simulink model "CARTESIAN_SPACE"  (R2018b)
settings: Solver=FixedStepAuto  StartTime=0.0  StopTime=25  FixedStep=0.01  RelTol=1e-3
model workspace: external: MATLAB File D:\OneDrive\STUDY\RIC LAB\PROJECT 6DOF\CODE\CODE 6DOF\06_TRAJECTORY PLANNING\02\ROBOT_DataFile.m (data not in the file)
undefined symbols (not defined in the file or in its folder): circle, smiData, X, Y, Z
libraries: sm_lib x38, nesl_utility x16, simulink_extras x1
(part 1 of 2)
settings Model: Creator=TMP  LastModifiedBy=TMP

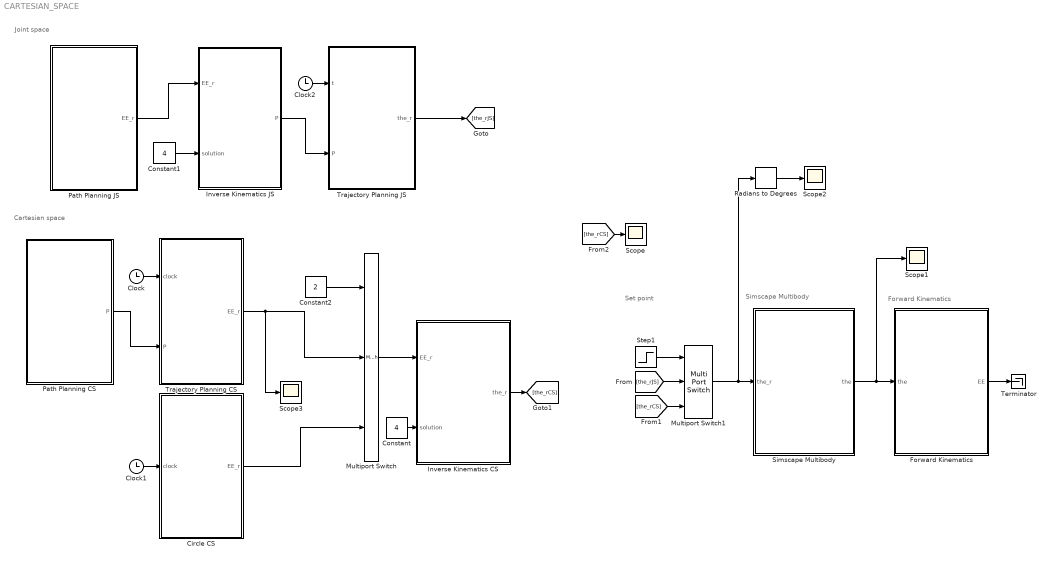
== system CARTESIAN_SPACE ==
  note: Set point
  note: Cartesian space
  note: Joint space
  note: Forward Kinematics
  note: Simscape Multibody
  Circle CS : MATLAB Function  TreatAsAtomicUnit=on
  Clock : Clock
  Clock1 : Clock
  Clock2 : Clock
  Constant : Constant  Value=4
  Constant1 : Constant  Value=4
  Constant2 : Constant  Value=2
  Forward Kinematics : MATLAB Function  TreatAsAtomicUnit=on
  Inverse Kinematics CS : MATLAB Function  TreatAsAtomicUnit=on
  Inverse Kinematics JS : MATLAB Function  TreatAsAtomicUnit=on
  Multiport Switch : MultiPortSwitch  Inputs=2
  Multiport Switch1 : MultiPortSwitch  Inputs=2
  Path Planning CS : Subsystem
  Path Planning JS : Subsystem
  Radians to Degrees : simulink_extras/Transformations/Radians to Degrees
  Scope{,1..3} (4 alike) : Scope
  Simscape Multibody : Subsystem
  Step1 : Step  Time=5  Before=1  After=2  SampleTime=0
  Terminator : Terminator
  Trajectory Planning CS : MATLAB Function  TreatAsAtomicUnit=on
  Trajectory Planning JS : MATLAB Function  TreatAsAtomicUnit=on
  wires:
  Clock1/1 -> Circle CS/1(clock)
  Circle CS/1(EE_r) -> Multiport Switch/3
  Constant/1 -> Inverse Kinematics CS/2(solution)
  Simscape Multibody/1(the) -> Scope1/1, Forward Kinematics/1(the)
  Multiport Switch/1 -> Inverse Kinematics CS/1(EE_r)
  Clock/1 -> Trajectory Planning CS/1(clock)
  Trajectory Planning CS/1(EE_r) -> Scope3/1, Multiport Switch/2
  Path Planning CS/1(P) -> Trajectory Planning CS/2(P)
  Constant2/1 -> Multiport Switch/1
  Clock2/1 -> Trajectory Planning JS/1(t)
  Path Planning JS/1(EE_r) -> Inverse Kinematics JS/1(EE_r)
  Constant1/1 -> Inverse Kinematics JS/2(solution)
  Inverse Kinematics JS/1(P) -> Trajectory Planning JS/2(P)
  Step1/1 -> Multiport Switch1/1
  Trajectory Planning JS/1(the_r) -> [the_rJS]
  Inverse Kinematics CS/1(the_r) -> [the_rCS]
  [the_rJS] -> Multiport Switch1/2
  [the_rCS] -> Multiport Switch1/3
  Forward Kinematics/1(EE) -> Terminator/1
  Multiport Switch1/1 -> Radians to Degrees/1, Simscape Multibody/1(the_r)
  [the_rCS] -> Scope/1
  Radians to Degrees/1 -> Scope2/1

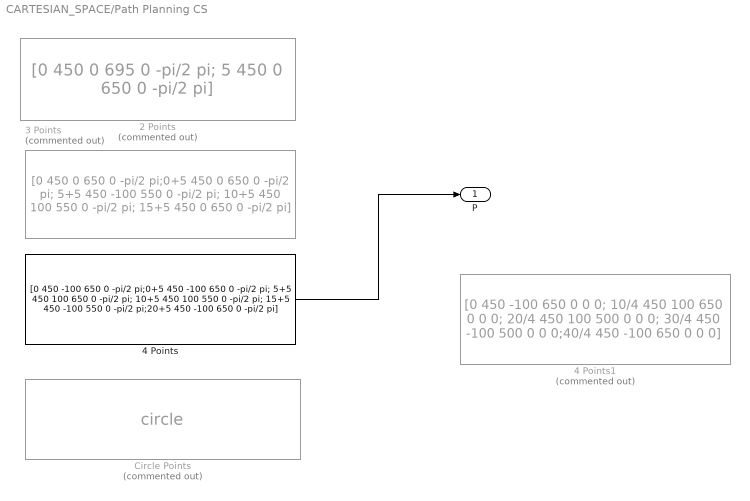
== system CARTESIAN_SPACE/Path Planning CS ==
  2 Points : Constant  Commented=on  Value=[0 450 0 695 0 -pi/2 pi; 5 450 0 650 0 -pi/2 pi]
  3 Points : Constant  Commented=on  Value=[0 450 0 650 0 -pi/2 pi;0+5 450 0 650 0 -pi/2 pi; 5+5 450 -100 550 0 -pi/2 pi; 10+5 450 100 550 0 -pi/2 pi; 15+5 450 0 650 0 -pi/2 pi]
  4 Points : Constant  Value=[0 450 -100 650 0 -pi/2 pi;0+5 450 -100 650 0 -pi/2 pi; 5+5 450 100 650 0 -pi/2 pi; 10+5 450 100 550 0 -pi/2 pi; 15+5 450 -100 550 0 -pi/2 pi;20+5 450 -100 650 0 -pi/2 pi]
  4 Points1 : Constant  Commented=on  Value=[0 450 -100 650 0 0 0; 10/4 450 100 650 0 0 0; 20/4 450 100 500 0 0 0; 30/4 450 -100 500 0 0 0;40/4 450 -100 650 0 0 0]
  Circle Points : Constant  Commented=on  Value=circle
  P : Outport
  wires:
  4 Points/1 -> P/1

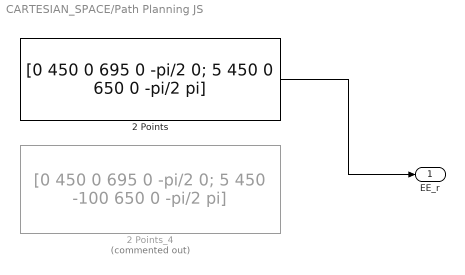
== system CARTESIAN_SPACE/Path Planning JS ==
  2 Points : Constant  Value=[0 450 0 695 0 -pi/2 0; 5 450 0 650 0 -pi/2 pi]
  2 Points_4 : Constant  Commented=on  Value=[0 450 0 695 0 -pi/2 0; 5 450 -100 650 0 -pi/2 pi]
  EE_r : Outport
  wires:
  2 Points/1 -> EE_r/1

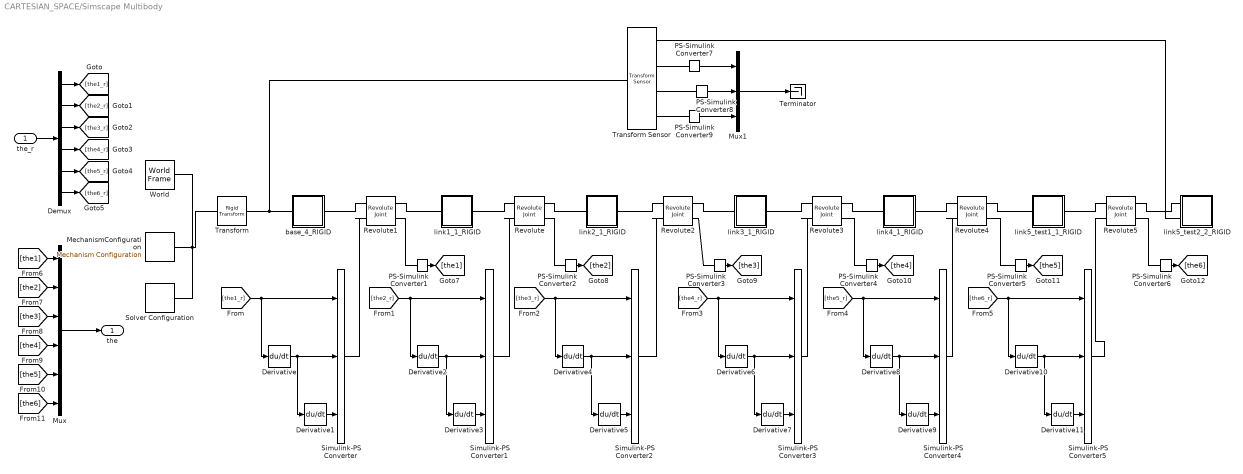
== system CARTESIAN_SPACE/Simscape Multibody ==
  the_r : Inport
  Demux : Demux  Outputs=6
  Derivative{,1..11} (12 alike) : Derivative
  MechanismConfiguration : sm_lib/Utilities/Mechanism Configuration  UniformGravity=Constant  GravityVector=[0 -9.80665 0]  GravityUnits=m/s^2  LinearizationDelta=0.001
  Mux : Mux  Inputs=6
  Mux1 : Mux  Inputs=3
  PS-Simulink Converter{1..9} (9 alike) : nesl_utility/PS-Simulink Converter  PhysicalDomain=network_engine_domain  SubClassName=ps_output  LeftPortType=input  RightPortType=output  PseudoPeriodic=off  Frequencies=[]  Unit=1  AffineConversion=off
  Revolute : sm_lib/Joints/Revolute Joint  SenseConstraintForce=off  SenseConstraintForceX=off  SenseConstraintForceY=off  SenseConstraintForceZ=off  SenseConstraintTorque=off  SenseConstraintTorqueX=off  SenseConstraintTorqueY=off  SenseConstraintTorqueZ=off  SenseTotalForce=off  SenseTotalForceX=off  SenseTotalForceY=off  SenseTotalForceZ=off  SenseTotalTorque=off  SenseTotalTorqueX=off  SenseTotalTorqueY=off  SenseTotalTorqueZ=off  CompositeWrenchDir=FollowerOnBase  CompositeWrenchFrame=BaseFrame  EquilibriumPosition=0  EquilibriumPositionUnits=rad  SpringStiffness=0  SpringStiffnessUnits=N*m/rad  DampingCoefficient=0  DampingCoefficientUnits=N*m/(rad/s)  TorqueActuationMode=ComputedTorque  MotionActuationMode=InputMotion  SensePosition=on  SenseVelocity=off  SenseAcceleration=off  SenseTorqueForce=off  PositionTargetSpecify=on  PositionTargetPriority=Low  PositionTargetValue=smiData.RevoluteJoint(1).Rz.Pos  PositionTargetValueUnits=deg  VelocityTargetSpecify=off  VelocityTargetPriority=High  VelocityTargetValue=0  VelocityTargetValueUnits=deg/s
  Revolute1 : sm_lib/Joints/Revolute Joint  SenseConstraintForce=off  SenseConstraintForceX=off  SenseConstraintForceY=off  SenseConstraintForceZ=off  SenseConstraintTorque=off  SenseConstraintTorqueX=off  SenseConstraintTorqueY=off  SenseConstraintTorqueZ=off  SenseTotalForce=off  SenseTotalForceX=off  SenseTotalForceY=off  SenseTotalForceZ=off  SenseTotalTorque=off  SenseTotalTorqueX=off  SenseTotalTorqueY=off  SenseTotalTorqueZ=off  CompositeWrenchDir=FollowerOnBase  CompositeWrenchFrame=BaseFrame  EquilibriumPosition=0  EquilibriumPositionUnits=rad  SpringStiffness=0  SpringStiffnessUnits=N*m/rad  DampingCoefficient=0  DampingCoefficientUnits=N*m/(rad/s)  TorqueActuationMode=ComputedTorque  MotionActuationMode=InputMotion  SensePosition=on  SenseVelocity=off  SenseAcceleration=off  SenseTorqueForce=off  PositionTargetSpecify=on  PositionTargetPriority=Low  PositionTargetValue=smiData.RevoluteJoint(2).Rz.Pos  PositionTargetValueUnits=deg  VelocityTargetSpecify=off  VelocityTargetPriority=High  VelocityTargetValue=0  VelocityTargetValueUnits=deg/s
  Revolute2 : sm_lib/Joints/Revolute Joint  SenseConstraintForce=off  SenseConstraintForceX=off  SenseConstraintForceY=off  SenseConstraintForceZ=off  SenseConstraintTorque=off  SenseConstraintTorqueX=off  SenseConstraintTorqueY=off  SenseConstraintTorqueZ=off  SenseTotalForce=off  SenseTotalForceX=off  SenseTotalForceY=off  SenseTotalForceZ=off  SenseTotalTorque=off  SenseTotalTorqueX=off  SenseTotalTorqueY=off  SenseTotalTorqueZ=off  CompositeWrenchDir=FollowerOnBase  CompositeWrenchFrame=BaseFrame  EquilibriumPosition=0  EquilibriumPositionUnits=rad  SpringStiffness=0  SpringStiffnessUnits=N*m/rad  DampingCoefficient=0  DampingCoefficientUnits=N*m/(rad/s)  TorqueActuationMode=ComputedTorque  MotionActuationMode=InputMotion  SensePosition=on  SenseVelocity=off  SenseAcceleration=off  SenseTorqueForce=off  PositionTargetSpecify=on  PositionTargetPriority=Low  PositionTargetValue=smiData.RevoluteJoint(3).Rz.Pos  PositionTargetValueUnits=deg  VelocityTargetSpecify=off  VelocityTargetPriority=High  VelocityTargetValue=0  VelocityTargetValueUnits=deg/s
  Revolute3 : sm_lib/Joints/Revolute Joint  SenseConstraintForce=off  SenseConstraintForceX=off  SenseConstraintForceY=off  SenseConstraintForceZ=off  SenseConstraintTorque=off  SenseConstraintTorqueX=off  SenseConstraintTorqueY=off  SenseConstraintTorqueZ=off  SenseTotalForce=off  SenseTotalForceX=off  SenseTotalForceY=off  SenseTotalForceZ=off  SenseTotalTorque=off  SenseTotalTorqueX=off  SenseTotalTorqueY=off  SenseTotalTorqueZ=off  CompositeWrenchDir=FollowerOnBase  CompositeWrenchFrame=BaseFrame  EquilibriumPosition=0  EquilibriumPositionUnits=rad  SpringStiffness=0  SpringStiffnessUnits=N*m/rad  DampingCoefficient=0  DampingCoefficientUnits=N*m/(rad/s)  TorqueActuationMode=ComputedTorque  MotionActuationMode=InputMotion  SensePosition=on  SenseVelocity=off  SenseAcceleration=off  SenseTorqueForce=off  PositionTargetSpecify=on  PositionTargetPriority=Low  PositionTargetValue=smiData.RevoluteJoint(4).Rz.Pos  PositionTargetValueUnits=deg  VelocityTargetSpecify=off  VelocityTargetPriority=High  VelocityTargetValue=0  VelocityTargetValueUnits=deg/s
  Revolute4 : sm_lib/Joints/Revolute Joint  SenseConstraintForce=off  SenseConstraintForceX=off  SenseConstraintForceY=off  SenseConstraintForceZ=off  SenseConstraintTorque=off  SenseConstraintTorqueX=off  SenseConstraintTorqueY=off  SenseConstraintTorqueZ=off  SenseTotalForce=off  SenseTotalForceX=off  SenseTotalForceY=off  SenseTotalForceZ=off  SenseTotalTorque=off  SenseTotalTorqueX=off  SenseTotalTorqueY=off  SenseTotalTorqueZ=off  CompositeWrenchDir=FollowerOnBase  CompositeWrenchFrame=BaseFrame  EquilibriumPosition=0  EquilibriumPositionUnits=rad  SpringStiffness=0  SpringStiffnessUnits=N*m/rad  DampingCoefficient=0  DampingCoefficientUnits=N*m/(rad/s)  TorqueActuationMode=ComputedTorque  MotionActuationMode=InputMotion  SensePosition=on  SenseVelocity=off  SenseAcceleration=off  SenseTorqueForce=off  PositionTargetSpecify=on  PositionTargetPriority=Low  PositionTargetValue=smiData.RevoluteJoint(5).Rz.Pos  PositionTargetValueUnits=deg  VelocityTargetSpecify=off  VelocityTargetPriority=High  VelocityTargetValue=0  VelocityTargetValueUnits=deg/s
  Revolute5 : sm_lib/Joints/Revolute Joint  SenseConstraintForce=off  SenseConstraintForceX=off  SenseConstraintForceY=off  SenseConstraintForceZ=off  SenseConstraintTorque=off  SenseConstraintTorqueX=off  SenseConstraintTorqueY=off  SenseConstraintTorqueZ=off  SenseTotalForce=off  SenseTotalForceX=off  SenseTotalForceY=off  SenseTotalForceZ=off  SenseTotalTorque=off  SenseTotalTorqueX=off  SenseTotalTorqueY=off  SenseTotalTorqueZ=off  CompositeWrenchDir=FollowerOnBase  CompositeWrenchFrame=BaseFrame  EquilibriumPosition=0  EquilibriumPositionUnits=rad  SpringStiffness=0  SpringStiffnessUnits=N*m/rad  DampingCoefficient=0  DampingCoefficientUnits=N*m/(rad/s)  TorqueActuationMode=ComputedTorque  MotionActuationMode=InputMotion  SensePosition=on  SenseVelocity=off  SenseAcceleration=off  SenseTorqueForce=off  PositionTargetSpecify=on  PositionTargetPriority=Low  PositionTargetValue=smiData.RevoluteJoint(6).Rz.Pos  PositionTargetValueUnits=deg  VelocityTargetSpecify=off  VelocityTargetPriority=High  VelocityTargetValue=0  VelocityTargetValueUnits=deg/s
  Simulink-PS Converter{,1..5} (6 alike) : nesl_utility/Simulink-PS Converter  PhysicalDomain=network_engine_domain  SubClassName=ps_input  LeftPortType=input  RightPortType=output  PseudoPeriodic=off  Frequencies=[]  NoiseDistribution=none  NoiseParameters=[]  Unit=1  AffineConversion=off  FilteringAndDerivatives=provide  SimscapeFilterOrder=1  InputFilterTimeConstant=0.001  UdotUserProvided=2
  Solver Configuration : nesl_utility/Solver Configuration  PhysicalDomain=network_engine_domain  SubClassName=solver  LeftPortType=input  RightPortType=generic  Tones=[]  Harmonics=[]  SimulateNoise=off  Profile=off  UseLocalSampling=off  EnableSwitchedLinearOptims=on  FrequencyDomain=off  UseCCode=off  RelTol=0.001  AbsTol=1e-06  MinStep=1e-09  ToWorkspace=off  RevertToSquareIcSolve=off  NumHomotopyIterations=100  PhasorMode=off  PhasorModeNumHarmonics=1  DoDC=off  ResidualTolerance=1e-09  UseLocalSolver=off  LocalSolverChoice=NE_BACKWARD_EULER_ADVANCER  LocalSolverSampleTime=0.001  DoFixedCost=off  MaxNonlinIter=3  MaxModeIter=2  LinearAlgebra=auto  EquationFormulation=NE_TIME_EF  DelaysMemoryBudget=1024  AutomaticFiltering=on  FilteringTimeConstant=0.001  PartitionStorageMethod=AS_NEEDED  PartitionMemoryBudget=1024
  Terminator : Terminator
  Transform : sm_lib/Frames and Transforms/Rigid Transform  TranslationMethod=Cartesian  TranslationStandardOffset=0  TranslationLengthUnit=m  TranslationStandardAxis=+Z  TranslationCartesianOffset=smiData.RigidTransform(13).translation  TranslationROffset=0  TranslationROffsetUnits=m  TranslationZOffset=0  TranslationZOffsetUnits=m  TranslationThetaOffset=0  TranslationThetaOffsetUnits=deg  RotationMethod=ArbitraryAxis  RotationAngleUnits=rad  RotationStandardAxis=+Z  RotationAngle=smiData.RigidTransform(13).angle  RotationArbitraryAxis=smiData.RigidTransform(13).axis  FollAlignAxisA=+X  BaseAlignAxisA=+Y  FollAlignAxisB=+Y  BaseAlignAxisB=+Z  RotationSequenceAxes=FollowerAxes  RotationSequence=XYX  RotationSequenceAngles=[0 0 0]  RotationSequenceAnglesUnits=deg  RotationMatrix=[1 0 0; 0 1 0; 0 0 1]
  Transform Sensor : sm_lib/Frames and Transforms/Transform Sensor  MeasurementFrame=World  SenseAngle=off  SenseAxis=off  SenseAngle1=off  SenseAngle2=off  SenseAngle3=off  SenseQ=off  SenseR=off  SenseOmegaX=off  SenseOmegaY=off  SenseOmegaZ=off  SenseOmega1=off  SenseOmega2=off  SenseOmega3=off  SenseQDot=off  SenseRDot=off  SenseAlphaX=off  SenseAlphaY=off  SenseAlphaZ=off  SenseAlpha1=off  SenseAlpha2=off  SenseAlpha3=off  SenseQDDot=off  SenseRDDot=off  SenseX=on  SenseY=on  SenseZ=on  SenseRad=off  SenseAzim=off  SenseDist=off  SenseInc=off  SenseXDot=off  SenseYDot=off  SenseZDot=off  SenseRadDot=off  SenseAzimDot=off  SenseDistDot=off  SenseIncDot=off  SenseXDDot=off  SenseYDDot=off  SenseZDDot=off  SenseRadDDot=off  SenseAzimDDot=off  SenseDistDDot=off  SenseIncDDot=off
  World : sm_lib/Frames and Transforms/World Frame
  base_4_RIGID : Subsystem
  link1_1_RIGID : Subsystem
  link2_1_RIGID : Subsystem
  link3_1_RIGID : Subsystem
  link4_1_RIGID : Subsystem
  link5_test1_1_RIGID : Subsystem
  link5_test2_2_RIGID : Subsystem
  the : Outport
  wires:
  [the3] -> Mux/3
  Demux/2 -> [the2_r]
  PS-Simulink Converter8/1 -> Mux1/2
  Derivative10/1 -> Simulink-PS Converter5/2, Derivative11/1
  PS-Simulink Converter7/1 -> Mux1/1
  Derivative6/1 -> Simulink-PS Converter3/2, Derivative7/1
  [the1_r] -> Derivative/1, Simulink-PS Converter/1
  [the6] -> Mux/6
  Derivative7/1 -> Simulink-PS Converter3/3
  PS-Simulink Converter9/1 -> Mux1/3
  Demux/6 -> [the6_r]
  [the5_r] -> Derivative8/1, Simulink-PS Converter4/1
  [the4_r] -> Simulink-PS Converter3/1, Derivative6/1
  Derivative1/1 -> Simulink-PS Converter/3
  PS-Simulink Converter1/1 -> [the1]
  the_r/1 -> Demux/1
  Mux/1 -> the/1
  PS-Simulink Converter5/1 -> [the5]
  PS-Simulink Converter2/1 -> [the2]
  [the4] -> Mux/4
  Derivative3/1 -> Simulink-PS Converter1/3
  [the5] -> Mux/5
  Demux/4 -> [the4_r]
  Demux/1 -> [the1_r]
  [the2] -> Mux/2
  [the3_r] -> Derivative4/1, Simulink-PS Converter2/1
  [the6_r] -> Simulink-PS Converter5/1, Derivative10/1
  Demux/5 -> [the5_r]
  Derivative4/1 -> Derivative5/1, Simulink-PS Converter2/2
  Derivative9/1 -> Simulink-PS Converter4/3
  [the1] -> Mux/1
  Demux/3 -> [the3_r]
  PS-Simulink Converter4/1 -> [the4]
  PS-Simulink Converter3/1 -> [the3]
  Derivative2/1 -> Simulink-PS Converter1/2, Derivative3/1
  Derivative8/1 -> Derivative9/1, Simulink-PS Converter4/2
  [the2_r] -> Simulink-PS Converter1/1, Derivative2/1
  PS-Simulink Converter6/1 -> [the6]
  Derivative/1 -> Derivative1/1, Simulink-PS Converter/2
  Derivative11/1 -> Simulink-PS Converter5/3
  Derivative5/1 -> Simulink-PS Converter2/3
  Mux1/1 -> Terminator/1
  connections:
  Revolute/LConn2 -- Simulink-PS Converter1/RConn1
  Revolute5/LConn1 -- link5_test1_1_RIGID/RConn1
  Revolute2/RConn1 -- link3_1_RIGID/LConn1
  Revolute1/LConn1 -- base_4_RIGID/RConn1
  Transform/LConn1 -- MechanismConfiguration/RConn1 -- Solver Configuration/RConn1 -- World/RConn1
  Revolute4/RConn1 -- link5_test1_1_RIGID/LConn1
  Revolute5/LConn2 -- Simulink-PS Converter5/RConn1
  PS-Simulink Converter9/LConn1 -- Transform Sensor/RConn4
  Revolute4/LConn2 -- Simulink-PS Converter4/RConn1
  PS-Simulink Converter8/LConn1 -- Transform Sensor/RConn3
  Revolute/LConn1 -- link1_1_RIGID/RConn1
  Revolute/RConn1 -- link2_1_RIGID/LConn1
  Revolute5/RConn1 -- link5_test2_2_RIGID/LConn1
  Revolute1/RConn1 -- link1_1_RIGID/LConn1
  PS-Simulink Converter5/LConn1 -- Revolute4/RConn2
  PS-Simulink Converter2/LConn1 -- Revolute/RConn2
  Revolute2/LConn1 -- link2_1_RIGID/RConn1
  Revolute3/LConn1 -- link3_1_RIGID/RConn1
  PS-Simulink Converter7/LConn1 -- Transform Sensor/RConn2
  Revolute3/RConn1 -- link4_1_RIGID/LConn1
  Transform/RConn1 -- Transform Sensor/LConn1 -- base_4_RIGID/LConn1
  Revolute4/LConn1 -- link4_1_RIGID/RConn1
  PS-Simulink Converter3/LConn1 -- Revolute2/RConn2
  Revolute2/LConn2 -- Simulink-PS Converter2/RConn1
  PS-Simulink Converter6/LConn1 -- Revolute5/RConn2
  PS-Simulink Converter1/LConn1 -- Revolute1/RConn2
  PS-Simulink Converter4/LConn1 -- Revolute3/RConn2
  Revolute1/LConn2 -- Simulink-PS Converter/RConn1
  Revolute3/LConn2 -- Simulink-PS Converter3/RConn1
  Transform Sensor/RConn1 -- link5_test2_2_RIGID/LConn2

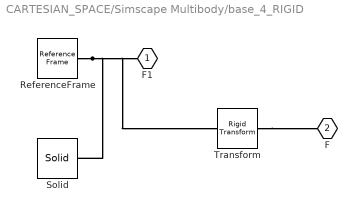
== system CARTESIAN_SPACE/Simscape Multibody/base_4_RIGID ==
  ReferenceFrame : sm_lib/Frames and Transforms/Reference Frame
  Solid : sm_lib/Body Elements/Solid  InertiaType=Custom  Mass=smiData.Solid(4).mass  MassUnits=kg  CenterOfMass=smiData.Solid(4).CoM  CenterOfMassUnits=m  MomentsOfInertia=smiData.Solid(4).MoI  MomentsOfInertiaUnits=kg*m^2  ProductsOfInertia=smiData.Solid(4).PoI  ProductsOfInertiaUnits=kg*m^2  BasedOnType=Density  Density=1000  DensityUnits=kg/m^3  DoExposeReferenceFrame=on  SerializedFrames=<Frames/>  GraphicType=FromGeometry  MarkerShape=Sphere  MarkerSize=10  GraphicVisPropType=SimpleVisualProperties  GraphicDiffuseColor=smiData.Solid(4).color  GraphicSpecularColor=[0.5 0.5 0.5 1.0]  GraphicAmbientColor=[0.15 0.15 0.15 1.0]  GraphicEmissiveColor=[0.0 0.0 0.0 1.0]  GraphicShininess=75  GraphicOpacity=smiData.Solid(4).opacity  GeometryShape=FromFile  RectangleSize=[1 1]  RectangleSizeUnits=m  BrickDimensions=[1 1 1]  BrickDimensionUnits=m  CylinderRadius=1  CylinderRadiusUnits=m  CylinderLength=1  CylinderLengthUnits=m  SphereRadius=1  SphereRadiusUnits=m  EllipsoidRadii=[1 1 1]  EllipsoidRadiiUnits=m  ExtrusionCrossSection=[1 1; -1 1; -1 -1; 1 -1]  ExtrusionCrossSectionUnits=m  ExtrusionLength=1  ExtrusionLengthUnits=m  PolygonNumSides=3  PolygonOuterRadius=1  PolygonOuterRadiusUnits=m  ExtGeomFileType=STEP  ExtGeomFileName=base_Default_sldprt.STEP  ExtGeomFileUnits=m  RevolutionCrossSection=[1 1; 1 -1; 2 -1; 2 1]  RevolutionCrossSectionUnits=m  RevolutionExtent=Full  RevolutionAngle=180  RevolutionAngleUnits=deg
  Transform : sm_lib/Frames and Transforms/Rigid Transform  TranslationMethod=Cartesian  TranslationStandardOffset=0  TranslationLengthUnit=m  TranslationStandardAxis=+Z  TranslationCartesianOffset=smiData.RigidTransform(3).translation  TranslationROffset=0  TranslationROffsetUnits=m  TranslationZOffset=0  TranslationZOffsetUnits=m  TranslationThetaOffset=0  TranslationThetaOffsetUnits=deg  RotationMethod=ArbitraryAxis  RotationAngleUnits=rad  RotationStandardAxis=+Z  RotationAngle=smiData.RigidTransform(3).angle  RotationArbitraryAxis=smiData.RigidTransform(3).axis  FollAlignAxisA=+X  BaseAlignAxisA=+Y  FollAlignAxisB=+Y  BaseAlignAxisB=+Z  RotationSequenceAxes=FollowerAxes  RotationSequence=XYX  RotationSequenceAngles=[0 0 0]  RotationSequenceAnglesUnits=deg  RotationMatrix=[1 0 0; 0 1 0; 0 0 1]
  F1 : PMIOPort  Side=Left
  F : PMIOPort  Port=2  Side=Right
  connections:
  Solid/RConn1 -- ReferenceFrame/RConn1 -- Transform/LConn1 -- F1/RConn1
  Transform/RConn1 -- F/RConn1

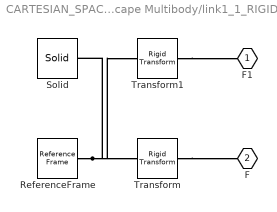
== system CARTESIAN_SPACE/Simscape Multibody/link1_1_RIGID ==
  ReferenceFrame : sm_lib/Frames and Transforms/Reference Frame
  Solid : sm_lib/Body Elements/Solid  InertiaType=Custom  Mass=smiData.Solid(7).mass  MassUnits=kg  CenterOfMass=smiData.Solid(7).CoM  CenterOfMassUnits=m  MomentsOfInertia=smiData.Solid(7).MoI  MomentsOfInertiaUnits=kg*m^2  ProductsOfInertia=smiData.Solid(7).PoI  ProductsOfInertiaUnits=kg*m^2  BasedOnType=Density  Density=1000  DensityUnits=kg/m^3  DoExposeReferenceFrame=on  SerializedFrames=<Frames/>  GraphicType=FromGeometry  MarkerShape=Sphere  MarkerSize=10  GraphicVisPropType=SimpleVisualProperties  GraphicDiffuseColor=smiData.Solid(7).color  GraphicSpecularColor=[0.5 0.5 0.5 1.0]  GraphicAmbientColor=[0.15 0.15 0.15 1.0]  GraphicEmissiveColor=[0.0 0.0 0.0 1.0]  GraphicShininess=75  GraphicOpacity=smiData.Solid(7).opacity  GeometryShape=FromFile  RectangleSize=[1 1]  RectangleSizeUnits=m  BrickDimensions=[1 1 1]  BrickDimensionUnits=m  CylinderRadius=1  CylinderRadiusUnits=m  CylinderLength=1  CylinderLengthUnits=m  SphereRadius=1  SphereRadiusUnits=m  EllipsoidRadii=[1 1 1]  EllipsoidRadiiUnits=m  ExtrusionCrossSection=[1 1; -1 1; -1 -1; 1 -1]  ExtrusionCrossSectionUnits=m  ExtrusionLength=1  ExtrusionLengthUnits=m  PolygonNumSides=3  PolygonOuterRadius=1  PolygonOuterRadiusUnits=m  ExtGeomFileType=STEP  ExtGeomFileName=link1_Default_sldprt.STEP  ExtGeomFileUnits=m  RevolutionCrossSection=[1 1; 1 -1; 2 -1; 2 1]  RevolutionCrossSectionUnits=m  RevolutionExtent=Full  RevolutionAngle=180  RevolutionAngleUnits=deg
  Transform : sm_lib/Frames and Transforms/Rigid Transform  TranslationMethod=Cartesian  TranslationStandardOffset=0  TranslationLengthUnit=m  TranslationStandardAxis=+Z  TranslationCartesianOffset=smiData.RigidTransform(1).translation  TranslationROffset=0  TranslationROffsetUnits=m  TranslationZOffset=0  TranslationZOffsetUnits=m  TranslationThetaOffset=0  TranslationThetaOffsetUnits=deg  RotationMethod=ArbitraryAxis  RotationAngleUnits=rad  RotationStandardAxis=+Z  RotationAngle=smiData.RigidTransform(1).angle  RotationArbitraryAxis=smiData.RigidTransform(1).axis  FollAlignAxisA=+X  BaseAlignAxisA=+Y  FollAlignAxisB=+Y  BaseAlignAxisB=+Z  RotationSequenceAxes=FollowerAxes  RotationSequence=XYX  RotationSequenceAngles=[0 0 0]  RotationSequenceAnglesUnits=deg  RotationMatrix=[1 0 0; 0 1 0; 0 0 1]
  Transform1 : sm_lib/Frames and Transforms/Rigid Transform  TranslationMethod=Cartesian  TranslationStandardOffset=0  TranslationLengthUnit=m  TranslationStandardAxis=+Z  TranslationCartesianOffset=smiData.RigidTransform(4).translation  TranslationROffset=0  TranslationROffsetUnits=m  TranslationZOffset=0  TranslationZOffsetUnits=m  TranslationThetaOffset=0  TranslationThetaOffsetUnits=deg  RotationMethod=ArbitraryAxis  RotationAngleUnits=rad  RotationStandardAxis=+Z  RotationAngle=smiData.RigidTransform(4).angle  RotationArbitraryAxis=smiData.RigidTransform(4).axis  FollAlignAxisA=+X  BaseAlignAxisA=+Y  FollAlignAxisB=+Y  BaseAlignAxisB=+Z  RotationSequenceAxes=FollowerAxes  RotationSequence=XYX  RotationSequenceAngles=[0 0 0]  RotationSequenceAnglesUnits=deg  RotationMatrix=[1 0 0; 0 1 0; 0 0 1]
  F1 : PMIOPort  Side=Left
  F : PMIOPort  Port=2  Side=Right
  connections:
  Solid/RConn1 -- ReferenceFrame/RConn1 -- Transform/LConn1 -- Transform1/LConn1
  Transform/RConn1 -- F/RConn1
  Transform1/RConn1 -- F1/RConn1

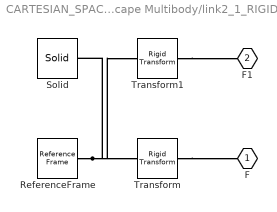
== system CARTESIAN_SPACE/Simscape Multibody/link2_1_RIGID ==
  ReferenceFrame : sm_lib/Frames and Transforms/Reference Frame
  Solid : sm_lib/Body Elements/Solid  InertiaType=Custom  Mass=smiData.Solid(3).mass  MassUnits=kg  CenterOfMass=smiData.Solid(3).CoM  CenterOfMassUnits=m  MomentsOfInertia=smiData.Solid(3).MoI  MomentsOfInertiaUnits=kg*m^2  ProductsOfInertia=smiData.Solid(3).PoI  ProductsOfInertiaUnits=kg*m^2  BasedOnType=Density  Density=1000  DensityUnits=kg/m^3  DoExposeReferenceFrame=on  SerializedFrames=<Frames/>  GraphicType=FromGeometry  MarkerShape=Sphere  MarkerSize=10  GraphicVisPropType=SimpleVisualProperties  GraphicDiffuseColor=smiData.Solid(3).color  GraphicSpecularColor=[0.5 0.5 0.5 1.0]  GraphicAmbientColor=[0.15 0.15 0.15 1.0]  GraphicEmissiveColor=[0.0 0.0 0.0 1.0]  GraphicShininess=75  GraphicOpacity=smiData.Solid(3).opacity  GeometryShape=FromFile  RectangleSize=[1 1]  RectangleSizeUnits=m  BrickDimensions=[1 1 1]  BrickDimensionUnits=m  CylinderRadius=1  CylinderRadiusUnits=m  CylinderLength=1  CylinderLengthUnits=m  SphereRadius=1  SphereRadiusUnits=m  EllipsoidRadii=[1 1 1]  EllipsoidRadiiUnits=m  ExtrusionCrossSection=[1 1; -1 1; -1 -1; 1 -1]  ExtrusionCrossSectionUnits=m  ExtrusionLength=1  ExtrusionLengthUnits=m  PolygonNumSides=3  PolygonOuterRadius=1  PolygonOuterRadiusUnits=m  ExtGeomFileType=STEP  ExtGeomFileName=link2_Default_sldprt.STEP  ExtGeomFileUnits=m  RevolutionCrossSection=[1 1; 1 -1; 2 -1; 2 1]  RevolutionCrossSectionUnits=m  RevolutionExtent=Full  RevolutionAngle=180  RevolutionAngleUnits=deg
  Transform : sm_lib/Frames and Transforms/Rigid Transform  TranslationMethod=Cartesian  TranslationStandardOffset=0  TranslationLengthUnit=m  TranslationStandardAxis=+Z  TranslationCartesianOffset=smiData.RigidTransform(2).translation  TranslationROffset=0  TranslationROffsetUnits=m  TranslationZOffset=0  TranslationZOffsetUnits=m  TranslationThetaOffset=0  TranslationThetaOffsetUnits=deg  RotationMethod=ArbitraryAxis  RotationAngleUnits=rad  RotationStandardAxis=+Z  RotationAngle=smiData.RigidTransform(2).angle  RotationArbitraryAxis=smiData.RigidTransform(2).axis  FollAlignAxisA=+X  BaseAlignAxisA=+Y  FollAlignAxisB=+Y  BaseAlignAxisB=+Z  RotationSequenceAxes=FollowerAxes  RotationSequence=XYX  RotationSequenceAngles=[0 0 0]  RotationSequenceAnglesUnits=deg  RotationMatrix=[1 0 0; 0 1 0; 0 0 1]
  Transform1 : sm_lib/Frames and Transforms/Rigid Transform  TranslationMethod=Cartesian  TranslationStandardOffset=0  TranslationLengthUnit=m  TranslationStandardAxis=+Z  TranslationCartesianOffset=smiData.RigidTransform(5).translation  TranslationROffset=0  TranslationROffsetUnits=m  TranslationZOffset=0  TranslationZOffsetUnits=m  TranslationThetaOffset=0  TranslationThetaOffsetUnits=deg  RotationMethod=ArbitraryAxis  RotationAngleUnits=rad  RotationStandardAxis=+Z  RotationAngle=smiData.RigidTransform(5).angle  RotationArbitraryAxis=smiData.RigidTransform(5).axis  FollAlignAxisA=+X  BaseAlignAxisA=+Y  FollAlignAxisB=+Y  BaseAlignAxisB=+Z  RotationSequenceAxes=FollowerAxes  RotationSequence=XYX  RotationSequenceAngles=[0 0 0]  RotationSequenceAnglesUnits=deg  RotationMatrix=[1 0 0; 0 1 0; 0 0 1]
  F : PMIOPort  Side=Left
  F1 : PMIOPort  Port=2  Side=Right
  connections:
  Solid/RConn1 -- ReferenceFrame/RConn1 -- Transform/LConn1 -- Transform1/LConn1
  Transform/RConn1 -- F/RConn1
  Transform1/RConn1 -- F1/RConn1

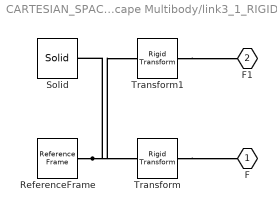
== system CARTESIAN_SPACE/Simscape Multibody/link3_1_RIGID ==
  ReferenceFrame : sm_lib/Frames and Transforms/Reference Frame
  Solid : sm_lib/Body Elements/Solid  InertiaType=Custom  Mass=smiData.Solid(2).mass  MassUnits=kg  CenterOfMass=smiData.Solid(2).CoM  CenterOfMassUnits=m  MomentsOfInertia=smiData.Solid(2).MoI  MomentsOfInertiaUnits=kg*m^2  ProductsOfInertia=smiData.Solid(2).PoI  ProductsOfInertiaUnits=kg*m^2  BasedOnType=Density  Density=1000  DensityUnits=kg/m^3  DoExposeReferenceFrame=on  SerializedFrames=<Frames/>  GraphicType=FromGeometry  MarkerShape=Sphere  MarkerSize=10  GraphicVisPropType=SimpleVisualProperties  GraphicDiffuseColor=smiData.Solid(2).color  GraphicSpecularColor=[0.5 0.5 0.5 1.0]  GraphicAmbientColor=[0.15 0.15 0.15 1.0]  GraphicEmissiveColor=[0.0 0.0 0.0 1.0]  GraphicShininess=75  GraphicOpacity=smiData.Solid(2).opacity  GeometryShape=FromFile  RectangleSize=[1 1]  RectangleSizeUnits=m  BrickDimensions=[1 1 1]  BrickDimensionUnits=m  CylinderRadius=1  CylinderRadiusUnits=m  CylinderLength=1  CylinderLengthUnits=m  SphereRadius=1  SphereRadiusUnits=m  EllipsoidRadii=[1 1 1]  EllipsoidRadiiUnits=m  ExtrusionCrossSection=[1 1; -1 1; -1 -1; 1 -1]  ExtrusionCrossSectionUnits=m  ExtrusionLength=1  ExtrusionLengthUnits=m  PolygonNumSides=3  PolygonOuterRadius=1  PolygonOuterRadiusUnits=m  ExtGeomFileType=STEP  ExtGeomFileName=link3_Default_sldprt.STEP  ExtGeomFileUnits=m  RevolutionCrossSection=[1 1; 1 -1; 2 -1; 2 1]  RevolutionCrossSectionUnits=m  RevolutionExtent=Full  RevolutionAngle=180  RevolutionAngleUnits=deg
  Transform : sm_lib/Frames and Transforms/Rigid Transform  TranslationMethod=Cartesian  TranslationStandardOffset=0  TranslationLengthUnit=m  TranslationStandardAxis=+Z  TranslationCartesianOffset=smiData.RigidTransform(6).translation  TranslationROffset=0  TranslationROffsetUnits=m  TranslationZOffset=0  TranslationZOffsetUnits=m  TranslationThetaOffset=0  TranslationThetaOffsetUnits=deg  RotationMethod=ArbitraryAxis  RotationAngleUnits=rad  RotationStandardAxis=+Z  RotationAngle=smiData.RigidTransform(6).angle  RotationArbitraryAxis=smiData.RigidTransform(6).axis  FollAlignAxisA=+X  BaseAlignAxisA=+Y  FollAlignAxisB=+Y  BaseAlignAxisB=+Z  RotationSequenceAxes=FollowerAxes  RotationSequence=XYX  RotationSequenceAngles=[0 0 0]  RotationSequenceAnglesUnits=deg  RotationMatrix=[1 0 0; 0 1 0; 0 0 1]
  Transform1 : sm_lib/Frames and Transforms/Rigid Transform  TranslationMethod=Cartesian  TranslationStandardOffset=0  TranslationLengthUnit=m  TranslationStandardAxis=+Z  TranslationCartesianOffset=smiData.RigidTransform(7).translation  TranslationROffset=0  TranslationROffsetUnits=m  TranslationZOffset=0  TranslationZOffsetUnits=m  TranslationThetaOffset=0  TranslationThetaOffsetUnits=deg  RotationMethod=ArbitraryAxis  RotationAngleUnits=rad  RotationStandardAxis=+Z  RotationAngle=smiData.RigidTransform(7).angle  RotationArbitraryAxis=smiData.RigidTransform(7).axis  FollAlignAxisA=+X  BaseAlignAxisA=+Y  FollAlignAxisB=+Y  BaseAlignAxisB=+Z  RotationSequenceAxes=FollowerAxes  RotationSequence=XYX  RotationSequenceAngles=[0 0 0]  RotationSequenceAnglesUnits=deg  RotationMatrix=[1 0 0; 0 1 0; 0 0 1]
  F : PMIOPort  Side=Left
  F1 : PMIOPort  Port=2  Side=Right
  connections:
  Solid/RConn1 -- ReferenceFrame/RConn1 -- Transform/LConn1 -- Transform1/LConn1
  Transform/RConn1 -- F/RConn1
  Transform1/RConn1 -- F1/RConn1

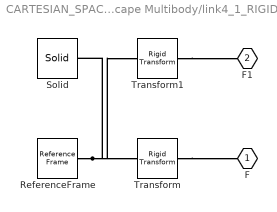
== system CARTESIAN_SPACE/Simscape Multibody/link4_1_RIGID ==
  ReferenceFrame : sm_lib/Frames and Transforms/Reference Frame
  Solid : sm_lib/Body Elements/Solid  InertiaType=Custom  Mass=smiData.Solid(5).mass  MassUnits=kg  CenterOfMass=smiData.Solid(5).CoM  CenterOfMassUnits=m  MomentsOfInertia=smiData.Solid(5).MoI  MomentsOfInertiaUnits=kg*m^2  ProductsOfInertia=smiData.Solid(5).PoI  ProductsOfInertiaUnits=kg*m^2  BasedOnType=Density  Density=1000  DensityUnits=kg/m^3  DoExposeReferenceFrame=on  SerializedFrames=<Frames/>  GraphicType=FromGeometry  MarkerShape=Sphere  MarkerSize=10  GraphicVisPropType=SimpleVisualProperties  GraphicDiffuseColor=smiData.Solid(5).color  GraphicSpecularColor=[0.5 0.5 0.5 1.0]  GraphicAmbientColor=[0.15 0.15 0.15 1.0]  GraphicEmissiveColor=[0.0 0.0 0.0 1.0]  GraphicShininess=75  GraphicOpacity=smiData.Solid(5).opacity  GeometryShape=FromFile  RectangleSize=[1 1]  RectangleSizeUnits=m  BrickDimensions=[1 1 1]  BrickDimensionUnits=m  CylinderRadius=1  CylinderRadiusUnits=m  CylinderLength=1  CylinderLengthUnits=m  SphereRadius=1  SphereRadiusUnits=m  EllipsoidRadii=[1 1 1]  EllipsoidRadiiUnits=m  ExtrusionCrossSection=[1 1; -1 1; -1 -1; 1 -1]  ExtrusionCrossSectionUnits=m  ExtrusionLength=1  ExtrusionLengthUnits=m  PolygonNumSides=3  PolygonOuterRadius=1  PolygonOuterRadiusUnits=m  ExtGeomFileType=STEP  ExtGeomFileName=link4_Default_sldprt.STEP  ExtGeomFileUnits=m  RevolutionCrossSection=[1 1; 1 -1; 2 -1; 2 1]  RevolutionCrossSectionUnits=m  RevolutionExtent=Full  RevolutionAngle=180  RevolutionAngleUnits=deg
  Transform : sm_lib/Frames and Transforms/Rigid Transform  TranslationMethod=Cartesian  TranslationStandardOffset=0  TranslationLengthUnit=m  TranslationStandardAxis=+Z  TranslationCartesianOffset=smiData.RigidTransform(8).translation  TranslationROffset=0  TranslationROffsetUnits=m  TranslationZOffset=0  TranslationZOffsetUnits=m  TranslationThetaOffset=0  TranslationThetaOffsetUnits=deg  RotationMethod=ArbitraryAxis  RotationAngleUnits=rad  RotationStandardAxis=+Z  RotationAngle=smiData.RigidTransform(8).angle  RotationArbitraryAxis=smiData.RigidTransform(8).axis  FollAlignAxisA=+X  BaseAlignAxisA=+Y  FollAlignAxisB=+Y  BaseAlignAxisB=+Z  RotationSequenceAxes=FollowerAxes  RotationSequence=XYX  RotationSequenceAngles=[0 0 0]  RotationSequenceAnglesUnits=deg  RotationMatrix=[1 0 0; 0 1 0; 0 0 1]
  Transform1 : sm_lib/Frames and Transforms/Rigid Transform  TranslationMethod=Cartesian  TranslationStandardOffset=0  TranslationLengthUnit=m  TranslationStandardAxis=+Z  TranslationCartesianOffset=smiData.RigidTransform(9).translation  TranslationROffset=0  TranslationROffsetUnits=m  TranslationZOffset=0  TranslationZOffsetUnits=m  TranslationThetaOffset=0  TranslationThetaOffsetUnits=deg  RotationMethod=ArbitraryAxis  RotationAngleUnits=rad  RotationStandardAxis=+Z  RotationAngle=smiData.RigidTransform(9).angle  RotationArbitraryAxis=smiData.RigidTransform(9).axis  FollAlignAxisA=+X  BaseAlignAxisA=+Y  FollAlignAxisB=+Y  BaseAlignAxisB=+Z  RotationSequenceAxes=FollowerAxes  RotationSequence=XYX  RotationSequenceAngles=[0 0 0]  RotationSequenceAnglesUnits=deg  RotationMatrix=[1 0 0; 0 1 0; 0 0 1]
  F : PMIOPort  Side=Left
  F1 : PMIOPort  Port=2  Side=Right
  connections:
  Solid/RConn1 -- ReferenceFrame/RConn1 -- Transform/LConn1 -- Transform1/LConn1
  Transform/RConn1 -- F/RConn1
  Transform1/RConn1 -- F1/RConn1

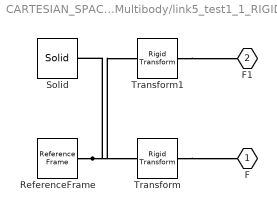
== system CARTESIAN_SPACE/Simscape Multibody/link5_test1_1_RIGID ==
  ReferenceFrame : sm_lib/Frames and Transforms/Reference Frame
  Solid : sm_lib/Body Elements/Solid  InertiaType=Custom  Mass=smiData.Solid(1).mass  MassUnits=kg  CenterOfMass=smiData.Solid(1).CoM  CenterOfMassUnits=m  MomentsOfInertia=smiData.Solid(1).MoI  MomentsOfInertiaUnits=kg*m^2  ProductsOfInertia=smiData.Solid(1).PoI  ProductsOfInertiaUnits=kg*m^2  BasedOnType=Density  Density=1000  DensityUnits=kg/m^3  DoExposeReferenceFrame=on  SerializedFrames=<Frames/>  GraphicType=FromGeometry  MarkerShape=Sphere  MarkerSize=10  GraphicVisPropType=SimpleVisualProperties  GraphicDiffuseColor=smiData.Solid(1).color  GraphicSpecularColor=[0.5 0.5 0.5 1.0]  GraphicAmbientColor=[0.15 0.15 0.15 1.0]  GraphicEmissiveColor=[0.0 0.0 0.0 1.0]  GraphicShininess=75  GraphicOpacity=smiData.Solid(1).opacity  GeometryShape=FromFile  RectangleSize=[1 1]  RectangleSizeUnits=m  BrickDimensions=[1 1 1]  BrickDimensionUnits=m  CylinderRadius=1  CylinderRadiusUnits=m  CylinderLength=1  CylinderLengthUnits=m  SphereRadius=1  SphereRadiusUnits=m  EllipsoidRadii=[1 1 1]  EllipsoidRadiiUnits=m  ExtrusionCrossSection=[1 1; -1 1; -1 -1; 1 -1]  ExtrusionCrossSectionUnits=m  ExtrusionLength=1  ExtrusionLengthUnits=m  PolygonNumSides=3  PolygonOuterRadius=1  PolygonOuterRadiusUnits=m  ExtGeomFileType=STEP  ExtGeomFileName=link5_test1_Default_sldprt.STEP  ExtGeomFileUnits=m  RevolutionCrossSection=[1 1; 1 -1; 2 -1; 2 1]  RevolutionCrossSectionUnits=m  RevolutionExtent=Full  RevolutionAngle=180  RevolutionAngleUnits=deg
  Transform : sm_lib/Frames and Transforms/Rigid Transform  TranslationMethod=Cartesian  TranslationStandardOffset=0  TranslationLengthUnit=m  TranslationStandardAxis=+Z  TranslationCartesianOffset=smiData.RigidTransform(10).translation  TranslationROffset=0  TranslationROffsetUnits=m  TranslationZOffset=0  TranslationZOffsetUnits=m  TranslationThetaOffset=0  TranslationThetaOffsetUnits=deg  RotationMethod=ArbitraryAxis  RotationAngleUnits=rad  RotationStandardAxis=+Z  RotationAngle=smiData.RigidTransform(10).angle  RotationArbitraryAxis=smiData.RigidTransform(10).axis  FollAlignAxisA=+X  BaseAlignAxisA=+Y  FollAlignAxisB=+Y  BaseAlignAxisB=+Z  RotationSequenceAxes=FollowerAxes  RotationSequence=XYX  RotationSequenceAngles=[0 0 0]  RotationSequenceAnglesUnits=deg  RotationMatrix=[1 0 0; 0 1 0; 0 0 1]
  Transform1 : sm_lib/Frames and Transforms/Rigid Transform  TranslationMethod=Cartesian  TranslationStandardOffset=0  TranslationLengthUnit=m  TranslationStandardAxis=+Z  TranslationCartesianOffset=smiData.RigidTransform(11).translation  TranslationROffset=0  TranslationROffsetUnits=m  TranslationZOffset=0  TranslationZOffsetUnits=m  TranslationThetaOffset=0  TranslationThetaOffsetUnits=deg  RotationMethod=ArbitraryAxis  RotationAngleUnits=rad  RotationStandardAxis=+Z  RotationAngle=smiData.RigidTransform(11).angle  RotationArbitraryAxis=smiData.RigidTransform(11).axis  FollAlignAxisA=+X  BaseAlignAxisA=+Y  FollAlignAxisB=+Y  BaseAlignAxisB=+Z  RotationSequenceAxes=FollowerAxes  RotationSequence=XYX  RotationSequenceAngles=[0 0 0]  RotationSequenceAnglesUnits=deg  RotationMatrix=[1 0 0; 0 1 0; 0 0 1]
  F : PMIOPort  Side=Left
  F1 : PMIOPort  Port=2  Side=Right
  connections:
  Solid/RConn1 -- ReferenceFrame/RConn1 -- Transform/LConn1 -- Transform1/LConn1
  Transform/RConn1 -- F/RConn1
  Transform1/RConn1 -- F1/RConn1

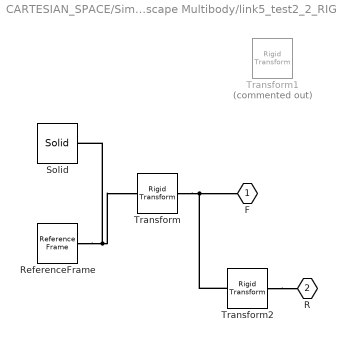
== system CARTESIAN_SPACE/Simscape Multibody/link5_test2_2_RIGID ==
  ReferenceFrame : sm_lib/Frames and Transforms/Reference Frame
  Solid : sm_lib/Body Elements/Solid  InertiaType=Custom  Mass=smiData.Solid(6).mass  MassUnits=kg  CenterOfMass=smiData.Solid(6).CoM  CenterOfMassUnits=m  MomentsOfInertia=smiData.Solid(6).MoI  MomentsOfInertiaUnits=kg*m^2  ProductsOfInertia=smiData.Solid(6).PoI  ProductsOfInertiaUnits=kg*m^2  BasedOnType=Density  Density=1000  DensityUnits=kg/m^3  DoExposeReferenceFrame=on  SerializedFrames=<Frames/>  GraphicType=FromGeometry  MarkerShape=Sphere  MarkerSize=10  GraphicVisPropType=SimpleVisualProperties  GraphicDiffuseColor=smiData.Solid(6).color  GraphicSpecularColor=[0.5 0.5 0.5 1.0]  GraphicAmbientColor=[0.15 0.15 0.15 1.0]  GraphicEmissiveColor=[0.0 0.0 0.0 1.0]  GraphicShininess=75  GraphicOpacity=smiData.Solid(6).opacity  GeometryShape=FromFile  RectangleSize=[1 1]  RectangleSizeUnits=m  BrickDimensions=[1 1 1]  BrickDimensionUnits=m  CylinderRadius=1  CylinderRadiusUnits=m  CylinderLength=1  CylinderLengthUnits=m  SphereRadius=1  SphereRadiusUnits=m  EllipsoidRadii=[1 1 1]  EllipsoidRadiiUnits=m  ExtrusionCrossSection=[1 1; -1 1; -1 -1; 1 -1]  ExtrusionCrossSectionUnits=m  ExtrusionLength=1  ExtrusionLengthUnits=m  PolygonNumSides=3  PolygonOuterRadius=1  PolygonOuterRadiusUnits=m  ExtGeomFileType=STEP  ExtGeomFileName=link5_test2_Default_sldprt.STEP  ExtGeomFileUnits=m  RevolutionCrossSection=[1 1; 1 -1; 2 -1; 2 1]  RevolutionCrossSectionUnits=m  RevolutionExtent=Full  RevolutionAngle=180  RevolutionAngleUnits=deg
  Transform : sm_lib/Frames and Transforms/Rigid Transform  TranslationMethod=Cartesian  TranslationStandardOffset=0  TranslationLengthUnit=m  TranslationStandardAxis=+Z  TranslationCartesianOffset=smiData.RigidTransform(12).translation  TranslationROffset=0  TranslationROffsetUnits=m  TranslationZOffset=0  TranslationZOffsetUnits=m  TranslationThetaOffset=0  TranslationThetaOffsetUnits=deg  RotationMethod=ArbitraryAxis  RotationAngleUnits=rad  RotationStandardAxis=+Z  RotationAngle=smiData.RigidTransform(12).angle  RotationArbitraryAxis=smiData.RigidTransform(12).axis  FollAlignAxisA=+X  BaseAlignAxisA=+Y  FollAlignAxisB=+Y  BaseAlignAxisB=+Z  RotationSequenceAxes=FollowerAxes  RotationSequence=XYX  RotationSequenceAngles=[0 0 0]  RotationSequenceAnglesUnits=deg  RotationMatrix=[1 0 0; 0 1 0; 0 0 1]
  Transform1 : sm_lib/Frames and Transforms/Rigid Transform  Commented=on  TranslationMethod=StandardAxis  TranslationStandardOffset=0.0006+0.0072092/1000  TranslationLengthUnit=m  TranslationStandardAxis=+Z  TranslationCartesianOffset=smiData.RigidTransform(12).translation  TranslationROffset=0  TranslationROffsetUnits=m  TranslationZOffset=0  TranslationZOffsetUnits=m  TranslationThetaOffset=0  TranslationThetaOffsetUnits=deg  RotationMethod=RotationSequence  RotationAngleUnits=rad  RotationStandardAxis=+Z  RotationAngle=smiData.RigidTransform(12).angle  RotationArbitraryAxis=smiData.RigidTransform(12).axis  FollAlignAxisA=+X  BaseAlignAxisA=+Y  FollAlignAxisB=+Y  BaseAlignAxisB=+Z  RotationSequenceAxes=FollowerAxes  RotationSequence=ZXZ  RotationSequenceAngles=[90 90 90]  RotationSequenceAnglesUnits=deg  RotationMatrix=[1 0 0; 0 1 0; 0 0 1]
  Transform2 : sm_lib/Frames and Transforms/Rigid Transform  TranslationMethod=StandardAxis  TranslationStandardOffset=0.038  TranslationLengthUnit=m  TranslationStandardAxis=+Z  TranslationCartesianOffset=smiData.RigidTransform(12).translation  TranslationROffset=0  TranslationROffsetUnits=m  TranslationZOffset=0  TranslationZOffsetUnits=m  TranslationThetaOffset=0  TranslationThetaOffsetUnits=deg  RotationMethod=None  RotationAngleUnits=rad  RotationStandardAxis=+Z  RotationAngle=smiData.RigidTransform(12).angle  RotationArbitraryAxis=smiData.RigidTransform(12).axis  FollAlignAxisA=+X  BaseAlignAxisA=+Y  FollAlignAxisB=+Y  BaseAlignAxisB=+Z  RotationSequenceAxes=FollowerAxes  RotationSequence=ZXZ  RotationSequenceAngles=[90 90 90]  RotationSequenceAnglesUnits=deg  RotationMatrix=[1 0 0; 0 1 0; 0 0 1]
  F : PMIOPort  Side=Left
  R : PMIOPort  Port=2  Side=Left
  connections:
  ReferenceFrame/RConn1 -- Solid/RConn1 -- Transform/LConn1
  Transform/RConn1 -- Transform2/LConn1 -- F/RConn1
  Transform2/RConn1 -- R/RConn1

== matlab function CARTESIAN_SPACE/Inverse Kinematics CS ==
  data: EE_r input; the_r output; solution input
function the_r  = IK_6DOF(EE_r,solution)
a1=75; a2=270; a3=90; d1=335; d4=295; d7=80;
emt = zeros(8,6);
m = 0;
px = EE_r(1);
py = EE_r(2);
pz = EE_r(3);
roll = EE_r(4);
pitch = EE_r(5);
yaw =  EE_r(6);
r11 = cos(yaw)*cos(pitch);
r21 = sin(yaw)*cos(pitch);
r31 = -sin(pitch);
r12 = cos(yaw)*sin(pitch)*sin(roll) - sin(yaw)*cos(roll);
r22 = sin(yaw)*sin(pitch)*sin(roll) + cos(yaw)*cos(roll);
r32 = cos(pitch)*sin(roll);
r13 = cos(yaw)*sin(pitch)*cos(roll) + sin(yaw)*sin(roll);
r23 = sin(yaw)*sin(pitch)*cos(roll) - cos(yaw)*sin(roll);
r33 = cos(pitch)*cos(roll);
% r11 = 1;
% r22 = 0;
% r33 = 0;
% r12 = 0;
% r21 = 0;
% r13 = 0;
% r31 = 0;
% r23 = -1;
% r32 = 1;
%% Inverse Kinematics
% Find the1
a_1 = py - r23*d7;
b_1 = - px + r13*d7;
d_1 = 0;
the11 = basic_01(a_1,b_1,d_1);
for i = 1:2
    % Find the2
    u = cos(the11(i))*(px-d7*r13) + sin(the11(i))*(py-r23*d7) - a1;
    v = pz - d1 - r33*d7;
    a_2 = v;
    b_2 = u;
    d_2 = (a3^2+d4^2-u^2-v^2-a2^2)/(-2*a2);
    if a_2*a_2 + b_2*b_2 - d_2*d_2 >=0
        the22 = basic_01(a_2,b_2,d_2);
    else
        continue;
    end
    for j = 1:2
        % Find the3
        a_3 = a3;
        b_3 = d4;
        c_3 = u*sin(the22(j)) + v*cos(the22(j)) - a2;
        d_3 = u*cos(the22(j)) - v*sin(the22(j));
        the33 = basic_02(a_3,b_3,c_3,d_3);
        
        % Find the5
        c5 = (r13*cos(the11(i))*cos(the22(j)) - r33*sin(the22(j)) + r23*cos(the22(j))*sin(the11(i)))*cos(the33) - (r33*cos(the22(j)) + r13*cos(the11(i))*sin(the22(j)) + r23*sin(the11(i))*sin(the22(j)))*sin(the33);
        if 1*1 + 0*0 - c5*c5 >=0
            the55 = basic_01(1,0,c5);
        else
            continue;
        end
        for k = 1:2
            % Find the4
            m = m+1;
            s4 = (r23*cos(the11(i)) - r13*sin(the11(i)))/(sin(the55(k)));
            c4 = (r33*cos(the22(j)) + r13*cos(the11(i))*sin(the22(j)) + r23*sin(the11(i))*sin(the22(j)) + sin(the33)*cos(the55(k))) / (-cos(the33)*sin(the55(k)));
            the44 = atan2(s4,c4);
            
            % Find the6
            a_6 = r21*cos(the11(i)) - r11*sin(the11(i));
            b_6 = r22*cos(the11(i)) - r12*sin(the11(i));
            c_6 = -sin(the44)*cos(the55(k));
            d_6 = cos(the44);
            the66 = basic_02(a_6,b_6,c_6,-d_6);
            emt(m,:)=[the11(i),the22(j),the33,the44,the55(k),the66];
        end
    end
end
% the = emt(solution,:);
the1 = emt(solution,1);
the2 = emt(solution,2);
the3 = emt(solution,3);
the4 = emt(solution,4);
the5 = emt(solution,5);
the6 = emt(solution,6);
the_r = [the1;the2;the3;the4;the5;the6];
end

function x = basic_01(a, b, d) % a*cos(x) + b*sin(x) = d
    anp = atan2(b, a);
    
    x1 = anp + atan2(sqrt(a*a + b*b - d*d), d);
    x2 = anp + atan2(-sqrt(a*a + b*b - d*d), d);
    x = [x1; x2];
end   

function x = basic_02(a, b, c, d) 
    % a*cos(x) - b*sin(x) = c
    % b*cos(x) + a*sin(x) = d
    sin = (d - b*c/a) / (b^2/a + a);
    cos = (c + b*d/a) / (b^2/a + a);
    x = atan2(sin,cos);
end

== matlab function CARTESIAN_SPACE/Forward Kinematics ==
  data: the input; EE output
function EE  = FK_6DOF(the)
the1 = the(1);
the2 = the(2);
the3 = the(3);
the4 = the(4);
the5 = the(5);
the6 = the(6);
a1=75; a2=270; a3=90; d1=335; d4=295; d7=80;

T_0_EE = ...
[ cos(the6)*(cos(the5)*sin(the1)*sin(the4) + cos(the2 + the3)*cos(the1)*sin(the5) + cos(the1)*cos(the2)*cos(the4)*cos(the5)*sin(the3) + cos(the1)*cos(the3)*cos(the4)*cos(the5)*sin(the2)) - sin(the6)*(cos(the1)*cos(the2)*sin(the3)*sin(the4) - cos(the4)*sin(the1) + cos(the1)*cos(the3)*sin(the2)*sin(the4)), - cos(the6)*(cos(the1)*cos(the2)*sin(the3)*sin(the4) - cos(the4)*sin(the1) + cos(the1)*cos(the3)*sin(the2)*sin(the4)) - sin(the6)*(cos(the5)*sin(the1)*sin(the4) + cos(the2 + the3)*cos(the1)*sin(the5) + cos(the1)*cos(the2)*cos(the4)*cos(the5)*sin(the3) + cos(the1)*cos(the3)*cos(the4)*cos(the5)*sin(the2)), cos(the2 + the3)*cos(the1)*cos(the5) - sin(the5)*(sin(the1)*sin(the4) + cos(the1)*cos(the2)*cos(the4)*sin(the3) + cos(the1)*cos(the3)*cos(the4)*sin(the2)), a1*cos(the1) + a2*cos(the1)*sin(the2) + d4*cos(the1)*cos(the2)*cos(the3) + a3*cos(the1)*cos(the2)*sin(the3) + a3*cos(the1)*cos(the3)*sin(the2) - d4*cos(the1)*sin(the2)*sin(the3) - d7*sin(the1)*sin(the4)*sin(the5) + d7*cos(the1)*cos(the2)*cos(the3)*cos(the5) - d7*cos(the1)*cos(the5)*sin(the2)*sin(the3) - d7*cos(the1)*cos(the2)*cos(the4)*sin(the3)*sin(the5) - d7*cos(the1)*cos(the3)*cos(the4)*sin(the2)*sin(the5);
  cos(the6)*(cos(the2 + the3)*sin(the1)*sin(the5) - cos(the1)*cos(the5)*sin(the4) + cos(the2)*cos(the4)*cos(the5)*sin(the1)*sin(the3) + cos(the3)*cos(the4)*cos(the5)*sin(the1)*sin(the2)) - sin(the6)*(cos(the1)*cos(the4) + cos(the2)*sin(the1)*sin(the3)*sin(the4) + cos(the3)*sin(the1)*sin(the2)*sin(the4)), - cos(the6)*(cos(the1)*cos(the4) + cos(the2)*sin(the1)*sin(the3)*sin(the4) + cos(the3)*sin(the1)*sin(the2)*sin(the4)) - sin(the6)*(cos(the2 + the3)*sin(the1)*sin(the5) - cos(the1)*cos(the5)*sin(the4) + cos(the2)*cos(the4)*cos(the5)*sin(the1)*sin(the3) + cos(the3)*cos(the4)*cos(the5)*sin(the1)*sin(the2)), cos(the2 + the3)*cos(the5)*sin(the1) - sin(the5)*(cos(the2)*cos(the4)*sin(the1)*sin(the3) - cos(the1)*sin(the4) + cos(the3)*cos(the4)*sin(the1)*sin(the2)), a1*sin(the1) + a2*sin(the1)*sin(the2) + d4*cos(the2)*cos(the3)*sin(the1) + a3*cos(the2)*sin(the1)*sin(the3) + a3*cos(the3)*sin(the1)*sin(the2) + d7*cos(the1)*sin(the4)*sin(the5) - d4*sin(the1)*sin(the2)*sin(the3) + d7*cos(the2)*cos(the3)*cos(the5)*sin(the1) - d7*cos(the5)*sin(the1)*sin(the2)*sin(the3) - d7*cos(the2)*cos(the4)*sin(the1)*sin(the3)*sin(the5) - d7*cos(the3)*cos(the4)*sin(the1)*sin(the2)*sin(the5);
                                                                                                                                                                                          - cos(the6)*(sin(the2 + the3)*sin(the5) - cos(the2 + the3)*cos(the4)*cos(the5)) - cos(the2 + the3)*sin(the4)*sin(the6),                                                                                                                                                                                             sin(the6)*(sin(the2 + the3)*sin(the5) - cos(the2 + the3)*cos(the4)*cos(the5)) - cos(the2 + the3)*cos(the6)*sin(the4),                                                                                        - sin(the2 + the3)*cos(the5) - cos(the2 + the3)*cos(the4)*sin(the5),                                                                                                                                        d1 + a2*cos(the2) + a3*cos(the2)*cos(the3) - d4*cos(the2)*sin(the3) - d4*cos(the3)*sin(the2) - a3*sin(the2)*sin(the3) - d7*cos(the2)*cos(the5)*sin(the3) - d7*cos(the3)*cos(the5)*sin(the2) - d7*cos(the2)*cos(the3)*cos(the4)*sin(the5) + d7*cos(the4)*sin(the2)*sin(the3)*sin(the5);
                                                                                                                                                                                                                                                                                                               0,                                                                                                                                                                                                                                                                                                                0,                                                                                                                                                          0,                                                                                                                                                                                                                                                                                                                                                                                                                            1];
 
r11 = T_0_EE(1,1);
r21 = T_0_EE(2,1);
r31 = T_0_EE(3,1);
r12 = T_0_EE(1,2);
r22 = T_0_EE(2,2);
r32 = T_0_EE(3,2);
r13 = T_0_EE(1,3);
r23 = T_0_EE(2,3);
r33 = T_0_EE(3,3);
pitch = atan2(-r31,sqrt(r11^2+r21^2));
if pitch == pi/2
    yaw = 0;
    roll = atan2(r12,r22);
elseif pitch == -pi/2
    yaw = 0;
    roll = -atan2(r12,r22) ;     
else
    yaw = atan2(r21/cos(pitch),r11/cos(pitch));
    roll = atan2(r32/cos(pitch),r33/cos(pitch));
end
Px = T_0_EE(1,4);
Py = T_0_EE(2,4);
Pz = T_0_EE(3,4);
EE = [Px,Py,Pz];
